simulink model "uub_test"  (R2015b)
settings: Solver=VariableStepAuto  StartTime=0.0  StopTime=10.0  RelTol=1e-3
settings Model: Creator=admin  LastModifiedBy=admin

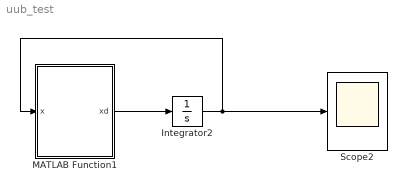
== system uub_test ==
  Integrator2 : Integrator  InitialCondition=10
  MATLAB Function1 : MATLAB Function  TreatAsAtomicUnit=on
  Scope2 : Scope
  wires:
  MATLAB Function1/1(xd) -> Integrator2/1
  Integrator2/1 -> MATLAB Function1/1(x), Scope2/1

== matlab function uub_test/MATLAB Function1 ==
  data: x input; xd output
function xd  = fcn(x)
%#codegen
c=100;
alpha=2;
xd=-alpha*x+c;
